simulink model "Simu_lab_6"  (R2020a)
settings: Solver=FixedStepAuto  StartTime=0.0  StopTime=10.0  FixedStep=1  RelTol=1e-3
settings Model: Creator=Miguel Gutierrez  LastModifiedBy=Miguel Gutierrez

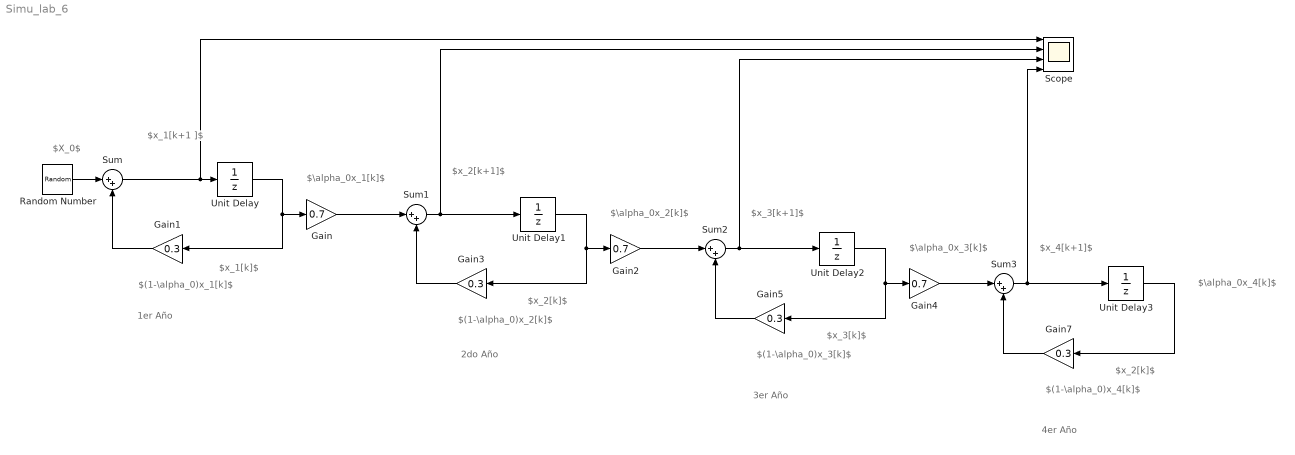
== system Simu_lab_6 ==
  note: 1er Año
  note: $X_0$
  note: $x_1[k]$
  note: $(1-\alpha_0)x_1[k]$
  note: $\alpha_0x_1[k]$
  note: 2do Año
  note: $x_1[k+1 ]$
  note: $x_2[k+1]$
  note: $\alpha_0x_2[k]$
  note: $x_2[k]$
  note: $(1-\alpha_0)x_2[k]$
  note: $(1-\alpha_0)x_3[k]$
  note: $x_3[k]$
  note: $\alpha_0x_3[k]$
  note: $x_3[k+1]$
  note: 3er Año
  note: 4er Año
  note: $(1-\alpha_0)x_4[k]$
  note: $x_4[k+1]$
  note: $\alpha_0x_4[k]$
  note: $x_2[k]$
  Gain : Gain  Gain=0.7
  Gain{1,3,5,7} (4 alike) : Gain  Gain=0.3
  Gain2 : Gain  Gain=0.7
  Gain4 : Gain  Gain=0.7
  Random Number : RandomNumber  Mean=25  Variance=4  SampleTime=1
  Scope : Scope  NumInputPorts=4
  Sum{,1..3} (4 alike) : Sum  Inputs=|++
  Unit Delay{,1..3} (4 alike) : UnitDelay  SampleTime=-1  HasFrameUpgradeWarning=on
  wires:
  Random Number/1 -> Sum/1
  Gain1/1 -> Sum/2
  Unit Delay/1 -> Gain/1, Gain1/1
  Sum/1 -> Scope/1, Unit Delay/1
  Unit Delay1/1 -> Gain2/1, Gain3/1
  Gain3/1 -> Sum1/2
  Gain/1 -> Sum1/1
  Unit Delay2/1 -> Gain4/1, Gain5/1
  Gain5/1 -> Sum2/2
  Gain2/1 -> Sum2/1
  Unit Delay3/1 -> Gain7/1
  Gain4/1 -> Sum3/1
  Gain7/1 -> Sum3/2
  Sum2/1 -> Scope/3, Unit Delay2/1
  Sum1/1 -> Unit Delay1/1, Scope/2
  Sum3/1 -> Unit Delay3/1, Scope/4
